simulink library "IAM_Table_KbL_KbT"  (Simulink 8.2)
settings: Solver=ode45  StartTime=0.0  StopTime=10.0  RelTol=1e-3
settings Model: Creator=lena.frank  LastModifiedBy=drhf

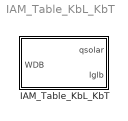
== system IAM_Table_KbL_KbT ==
  IAM_Table_KbL_KbT : Subsystem  mask(IAM Table for EN 12975 Solar Thermal Collector Model){fta=0.8, kblangle=[0:5:90], KbL=[1.0000    1.0000    0.9999    0.9996    0.9991    0.9982    0.9965  0.9935    0.9886    0.9807    0.9678    0.9473    0.9148    0.8638   0.7846    0.6644    0.4907    0.2599    0.0000], kbtangle=[0:5:90], KbT=[1.00000 1.00000 1.00000 1.00000 1.00000 1.00000 1.00000 1.00000 1.00000 1.00000 1.00000 0.87500 0.75000 0.62500 0.50000 0.37500 0.25000 0.12500 0], Kd=0.92}
      mask prompts: fta "Fin Efficiency * Transmission * Absorption (F'(tau alfa))"; kblangle "KbL: angles for longitudinal IAM [degree]"; KbL "KbL: values for longitudinal incidence angle modifier (0..1)"; kbtangle "KbT: angles for transversal IAM [degree]"; KbT "KbT: values for transversal incidence angle modifier (0..1)"; Kd "Kd : Incidence angle modifier diffuse radiation"
      mask help:
      | USE IN THE "Collector_EN12975" MODEL:
      | Transforms direct and diffuse radiation to an absorbed solar power per unit area. The direct radiation incidence angle modifier (Kdir) uses the b0-model for flat plate collectors (EN 12975).
      | FTA or F'(TauAlfa) is defined from the incidence angle modifiers Kdir and Kdfu:
      | FTA = eta0 / (Kdir(15°)*0.85 + Kdfu*0.15)
      | The direct radiation is split in a transversal (T) and longitudinal (L) component.
      | Direct radiation: Kb(L) and Kb(T) is given in an vecorized form
      | Diffuse radiation  Kd = constant (at 50° incidence)
      mask Help: web(fullfile(path_carnot('help'),'IAM_Table_KbL_KbT.html'),'-helpbrowser')

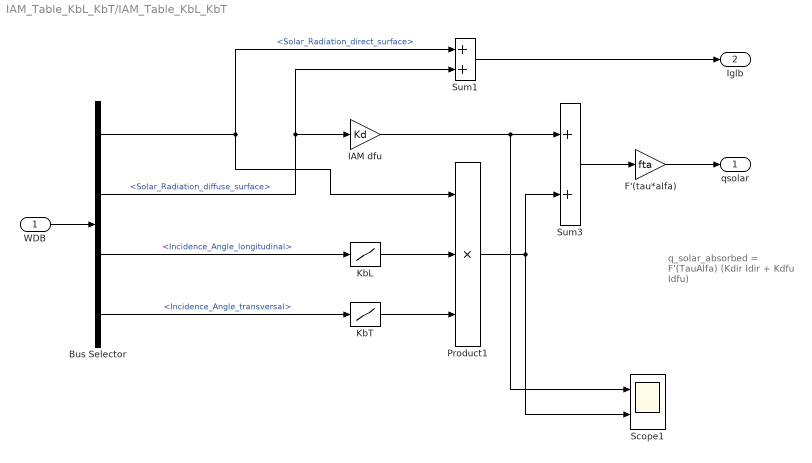
== system IAM_Table_KbL_KbT/IAM_Table_KbL_KbT ==
  note: q_solar_absorbed = F'(TauAlfa) (Kdir Idir + Kdfu Idfu)
  WDB : Inport
  Bus Selector : BusSelector  OutputSignals=Solar_Radiation_direct_surface,Solar_Radiation_diffuse_surface,Incidence_Angle_longitudinal,Incidence_Angle_transversal
  F'(tau*alfa) : Gain  Gain=fta  SaturateOnIntegerOverflow=on  OutDataTypeStr=Inherit: Same as input  ParamDataTypeStr=Inherit: Same as input
  IAM dfu : Gain  Gain=Kd  SaturateOnIntegerOverflow=on  OutDataTypeStr=Inherit: Same as input  ParamDataTypeStr=Inherit: Same as input
  KbL : Lookup  InputValues=kblangle  Table=KbL  SaturateOnIntegerOverflow=on
  KbT : Lookup  InputValues=kbtangle  Table=KbT  SaturateOnIntegerOverflow=on
  Product1 : Product  Inputs=3  SaturateOnIntegerOverflow=on  InputSameDT=on  OutDataTypeStr=Inherit: Same as first input
  Scope1 : Scope  NumInputPorts=2
      settings: YMin=-5~-5  YMax=5~5  SaveName=ScopeData2
  Sum1 : Sum  SaturateOnIntegerOverflow=on  InputSameDT=on  OutDataTypeStr=Inherit: Same as first input
  Sum3 : Sum  SaturateOnIntegerOverflow=on  InputSameDT=on  OutDataTypeStr=Inherit: Same as first input
  qsolar : Outport
  Iglb : Outport  Port=2
  wires:
  WDB/1 -> Bus Selector/1
  Product1/1 -> Sum3/2, Scope1/2
  Bus Selector/1 -> Sum1/1, Product1/1  "<Solar_Radiation_direct_surface>"
  Bus Selector/2 -> Sum1/2, IAM dfu/1  "<Solar_Radiation_diffuse_surface>"
  Bus Selector/4 -> KbT/1  "<Incidence_Angle_transversal>"
  Bus Selector/3 -> KbL/1  "<Incidence_Angle_longitudinal>"
  KbL/1 -> Product1/2
  KbT/1 -> Product1/3
  Sum3/1 -> F'(tau*alfa)/1
  Sum1/1 -> Iglb/1
  F'(tau*alfa)/1 -> qsolar/1
  IAM dfu/1 -> Sum3/1, Scope1/1
